simulink model "lab22"  (Simulink 6.0)
settings: Solver=ode45  StartTime=0.0  StopTime=10.0  RelTol=1e-3
settings Model: LastModifiedBy=student

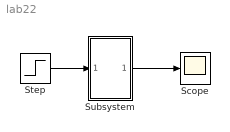
== system lab22 ==
  Scope : Scope
  Step : Step  Time=0  SampleTime=0
  Subsystem : Subsystem  mask{a=12}
      mask CallbackString:
      | if str2num(get_param(gcb,'a'))<0
      | 	error('panta este negativa')
      | end
  wires:
  Step/1 -> Subsystem/1(In1)
  Subsystem/1(Out1) -> Scope/1

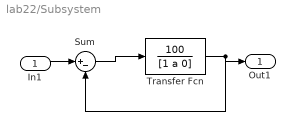
== system lab22/Subsystem ==
  In1 : Inport  Port=1  LatchInput=off
  Sum : Sum  Inputs=|+-
  Transfer Fcn : TransferFcn  Numerator=[100]  Denominator=[1 a 0]
  Out1 : Outport
  wires:
  Sum/1 -> Transfer Fcn/1
  Transfer Fcn/1 -> Sum/2, Out1/1
  In1/1 -> Sum/1
